simulink library "TM_DynamicModel_Library"  (Simulink 7.8)
settings: Solver=ode45  StartTime=0.0  StopTime=10.0  RelTol=1e-3
undefined symbols (not defined in the file or in its folder): DiscIntNeverNeededParam
libraries: simulink x43, TM_DynamicModel_Library x7
(part 2 of 2)

== system TM_DynamicModel_Library/DM_Eprec_FlgPreCdngAcvMod ==
  Constant : Constant  Value=0
  Eprec_FlgPreCdngAcvMod : Outport
  wires:
  Constant/1 -> Eprec_FlgPreCdngAcvMod/1

== system TM_DynamicModel_Library/DM_Err_ECT_low ==
  Constant : Constant  Value=0
  Err_ECT_low : Outport
  wires:
  Constant/1 -> Err_ECT_low/1

== system TM_DynamicModel_Library/DM_Esig_BmsTpMax ==
  Bms48_Tp : Inport
  Constant : Constant
  Sum : Sum  Inputs=|++
  Esig_BmsTpMax : Outport
  wires:
  Bms48_Tp/1 -> Sum/1
  Sum/1 -> Esig_BmsTpMax/1
  Constant/1 -> Sum/2

== system TM_DynamicModel_Library/DM_Esig_BmsTpMin ==
  Bms48_Tp : Inport
  Constant : Constant
  Sum1 : Sum  Inputs=|-+
  Esig_BmsTpMin : Outport
  wires:
  Bms48_Tp/1 -> Sum1/2
  Constant/1 -> Sum1/1
  Sum1/1 -> Esig_BmsTpMin/1

== system TM_DynamicModel_Library/DM_Esig_BmsTpTar ==
  Constant : Constant  Value=28
  Esig_BmsTpTar : Outport
  wires:
  Constant/1 -> Esig_BmsTpTar/1

== system TM_DynamicModel_Library/DM_FRT_Sens ==
  Constant : Constant  Value=25
  FRT_Sens : Outport
  wires:
  Constant/1 -> FRT_Sens/1

== system TM_DynamicModel_Library/DM_FirstStrt_Mode ==
  Constant : Constant  Value=0
  FirstStrt_Mode : Outport
  wires:
  Constant/1 -> FirstStrt_Mode/1

== system TM_DynamicModel_Library/DM_FirstStrt_Mode_EE ==
  Constant : Constant  Value=0
  FirstStrt_Mode_EE : Outport
  wires:
  Constant/1 -> FirstStrt_Mode_EE/1

== system TM_DynamicModel_Library/DM_Fuel_Temp ==
  Constant : Constant  Value=25
  Fuel_Temp : Outport
  wires:
  Constant/1 -> Fuel_Temp/1

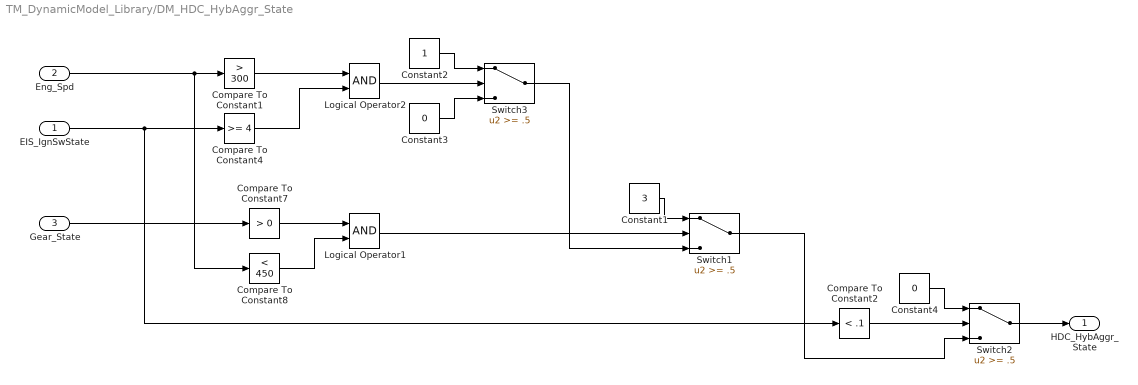
== system TM_DynamicModel_Library/DM_HDC_HybAggr_State ==
  EIS_IgnSwState : Inport
  Eng_Spd : Inport  Port=2
  Gear_State : Inport  Port=3
  Compare To Constant1 : simulink/Logic and Bit Operations/Compare To Constant  relop=>  const=300  OutDataTypeStr=uint8
  Compare To Constant2 : simulink/Logic and Bit Operations/Compare To Constant  relop=<  const=.1  OutDataTypeStr=uint8
  Compare To Constant4 : simulink/Logic and Bit Operations/Compare To Constant  relop=>=  const=4  OutDataTypeStr=uint8
  Compare To Constant7 : simulink/Logic and Bit Operations/Compare To Constant  relop=>  const=0  OutDataTypeStr=uint8
  Compare To Constant8 : simulink/Logic and Bit Operations/Compare To Constant  relop=<  const=450  OutDataTypeStr=uint8
  Constant1 : Constant  Value=3
  Constant2 : Constant
  Constant3 : Constant  Value=0
  Constant4 : Constant  Value=0
  Logical Operator1 : Logic  AllPortsSameDT=off  OutDataTypeStr=boolean
  Logical Operator2 : Logic  AllPortsSameDT=off  OutDataTypeStr=boolean
  Switch1 : Switch  Threshold=.5
  Switch2 : Switch  Threshold=.5
  Switch3 : Switch  Threshold=.5
  HDC_HybAggr_State : Outport
  wires:
  Gear_State/1 -> Compare To Constant7/1
  Eng_Spd/1 -> Compare To Constant8/1, Compare To Constant1/1
  EIS_IgnSwState/1 -> Compare To Constant4/1, Compare To Constant2/1
  Compare To Constant1/1 -> Logical Operator2/1
  Compare To Constant4/1 -> Logical Operator2/2
  Constant2/1 -> Switch3/1
  Constant3/1 -> Switch3/3
  Logical Operator2/1 -> Switch3/2
  Compare To Constant7/1 -> Logical Operator1/1
  Compare To Constant8/1 -> Logical Operator1/2
  Logical Operator1/1 -> Switch1/2
  Constant1/1 -> Switch1/1
  Switch3/1 -> Switch1/3
  Compare To Constant2/1 -> Switch2/2
  Switch1/1 -> Switch2/3
  Switch2/1 -> HDC_HybAggr_State/1
  Constant4/1 -> Switch2/1

== system TM_DynamicModel_Library/DM_HDC_HybSync_State ==
  Eng_Spd : Inport
  Eng_Trq : Inport  Port=2
  Add : Sum
  Add1 : Sum  Inputs=+-
  Add2 : Sum  Inputs=+-
  Constant : Constant  Value=13
  Constant1 : Constant  Value=31
  Constant2 : Constant  Value=0
  Constant3 : Constant  Value=0
  DM_AGC_ASSStop_Mode : TM_DynamicModel_Library/DM_AGC_ASSStop_Mode
  Switch : Switch  Threshold=1
  Switch1 : Switch  Threshold=1
  Unit Delay : UnitDelay  SampleTime=-1
  Unit Delay1 : UnitDelay  SampleTime=-1
  HDC_HybSync_State : Outport
  wires:
  Constant1/1 -> Switch1/1
  Constant2/1 -> Switch1/3
  Switch/1 -> Add/1
  Switch1/1 -> Add/2
  Add/1 -> HDC_HybSync_State/1
  Unit Delay/1 -> Add1/2
  Constant/1 -> Switch/1
  Constant3/1 -> Switch/3
  Add1/1 -> Switch/2
  Unit Delay1/1 -> Add2/1
  Add2/1 -> Switch1/2
  DM_AGC_ASSStop_Mode/1 -> Unit Delay/1, Add1/1, Unit Delay1/1, Add2/2
  Eng_Spd/1 -> DM_AGC_ASSStop_Mode/1
  Eng_Trq/1 -> DM_AGC_ASSStop_Mode/2

== system TM_DynamicModel_Library/DM_HDC_PTReady_Mode ==
  Eng_Spd : Inport
  EIS_IgnSwState : Inport  Port=2
  Compare To Constant : simulink/Logic and Bit Operations/Compare To Constant  relop=<  const=100  OutDataTypeStr=uint8
  Compare To Constant1 : simulink/Logic and Bit Operations/Compare To Constant  relop=>  const=3  OutDataTypeStr=uint8
  Constant : Constant  Value=0
  Constant1 : Constant
  DM_Ign_Mode : Subsystem
  Logical Operator1 : Logic  Operator=OR  Inputs=3  AllPortsSameDT=off  OutDataTypeStr=boolean
  Logical Operator2 : Logic  Operator=NOT  AllPortsSameDT=off  OutDataTypeStr=boolean
  Logical Operator3 : Logic  Operator=NOT  AllPortsSameDT=off  OutDataTypeStr=boolean
  Switch : Switch  Criteria=u2 > Threshold
  HDC_PTReady_Mode : Outport
  wires:
  Eng_Spd/1 -> Compare To Constant/1  "Eng_Spd"
  EIS_IgnSwState/1 -> Compare To Constant1/1, DM_Ign_Mode/1(EIS_IgnSwState)  "EIS_IgnSwState"
  Logical Operator2/1 -> Logical Operator1/2
  Compare To Constant1/1 -> Logical Operator3/1  "IgnSwCAN_Mode"
  Logical Operator3/1 -> Logical Operator1/3
  Switch/1 -> HDC_PTReady_Mode/1
  Logical Operator1/1 -> Switch/2
  Constant1/1 -> Switch/3
  Constant/1 -> Switch/1
  Compare To Constant/1 -> Logical Operator1/1
  DM_Ign_Mode/1(Ign_Mode) -> Logical Operator2/1

== system TM_DynamicModel_Library/DM_HVAC_CoolVlv_Rq ==
  Constant : Constant  Value=0
  HVAC_CoolVlv_Rq : Outport
  wires:
  Constant/1 -> HVAC_CoolVlv_Rq/1

== system TM_DynamicModel_Library/DM_Hepm_PwrMax48VEcm ==
  Constant : Constant  Value=7000
  Hepm_PwrMax48VEcm : Outport
  wires:
  Constant/1 -> Hepm_PwrMax48VEcm/1

== system TM_DynamicModel_Library/DM_Hpmc_StPlgnOpmdDispd ==
  Constant : Constant  Value=3
  Hpmc_StPlgnOpmdDispd : Outport
  wires:
  Constant/1 -> Hpmc_StPlgnOpmdDispd/1

== system TM_DynamicModel_Library/DM_HvacChil_ExpVlvPosnReq ==
  Constant : Constant  Value=0
  HvacChil_ExpVlvPosnReq : Outport
  wires:
  Constant/1 -> HvacChil_ExpVlvPosnReq/1

== system TM_DynamicModel_Library/DM_Hvac_StDefrstAcv ==
  Constant : Constant  Value=0
  Hvac_StDefrstAcv : Outport
  wires:
  Constant/1 -> Hvac_StDefrstAcv/1

== system TM_DynamicModel_Library/DM_IC_Knk_Red_Avg ==
  Constant : Constant  Value=0
  IC_Knk_Red_Avg : Outport
  wires:
  Constant/1 -> IC_Knk_Red_Avg/1

== system TM_DynamicModel_Library/DM_IC_Knk_Red_Avg_Actv ==
  Constant : Constant  Value=0
  IC_Knk_Red_Avg_Actv : Outport
  wires:
  Constant/1 -> IC_Knk_Red_Avg_Actv/1

== system TM_DynamicModel_Library/DM_Idle_Mode_Req ==
  APP : Inport
  Compare To Constant : simulink/Logic and Bit Operations/Compare To Constant  relop=<=  const=3.2  OutDataTypeStr=uint8
  DM_APP_Char_out_ub : Subsystem
  Data Type Conversion : DataTypeConversion
  Idle_Mode_Req : Outport
  wires:
  Data Type Conversion/1 -> Idle_Mode_Req/1
  Compare To Constant/1 -> Data Type Conversion/1
  DM_APP_Char_out_ub/1(APP_Char_out_ub) -> Compare To Constant/1
  APP/1 -> DM_APP_Char_out_ub/1(APP)

== system TM_DynamicModel_Library/DM_IgnSwRun_Mode ==
  EIS_IgnSwState : Inport
  Constant : Constant  Value=4
  Relational Operator : RelationalOperator  Operator===  OutDataTypeStr=boolean
  IgnSwRun_Mode : Outport
  wires:
  Constant/1 -> Relational Operator/2
  EIS_IgnSwState/1 -> Relational Operator/1
  Relational Operator/1 -> IgnSwRun_Mode/1  "IgnSwRun_Mode"

== system TM_DynamicModel_Library/DM_IgnSwStrtr_Mode ==
  EIS_IgnSwState : Inport
  Compare To Constant : simulink/Logic and Bit Operations/Compare To Constant  relop=>  const=4  OutDataTypeStr=uint8
  Compare To Constant1 : simulink/Logic and Bit Operations/Compare To Constant  relop=<  const=6  OutDataTypeStr=uint8
  Data Type Conversion : DataTypeConversion
  Logical Operator : Logic  AllPortsSameDT=off  OutDataTypeStr=boolean
  IgnSwStrtr_Mode : Outport
  wires:
  Data Type Conversion/1 -> IgnSwStrtr_Mode/1
  EIS_IgnSwState/1 -> Compare To Constant/1, Compare To Constant1/1
  Compare To Constant1/1 -> Logical Operator/2
  Compare To Constant/1 -> Logical Operator/1
  Logical Operator/1 -> Data Type Conversion/1

== system TM_DynamicModel_Library/DM_Ign_Mode ==
  EIS_IgnSwState : Inport
  Constant : Constant  Value=3
  Data Type Conversion : DataTypeConversion
  Relational Operator : RelationalOperator  OutDataTypeStr=boolean
  Ign_Mode : Outport
  wires:
  Data Type Conversion/1 -> Ign_Mode/1
  Constant/1 -> Relational Operator/2
  EIS_IgnSwState/1 -> Relational Operator/1
  Relational Operator/1 -> Data Type Conversion/1

== system TM_DynamicModel_Library/DM_Injr_Tp ==
  Constant : Constant  Value=25
  Injr_Tp : Outport
  wires:
  Constant/1 -> Injr_Tp/1

== system TM_DynamicModel_Library/DM_K15 ==
  EIS_IgnSwState : Inport
  Constant : Constant  Value=2
  Data Type Conversion : DataTypeConversion
  Data Type Conversion1 : DataTypeConversion  OutDataTypeStr=uint8
  Relational Operator : RelationalOperator  Operator=>  OutDataTypeStr=boolean
  K15 : Outport
  wires:
  Data Type Conversion1/1 -> Relational Operator/1
  Data Type Conversion/1 -> K15/1
  EIS_IgnSwState/1 -> Data Type Conversion1/1
  Constant/1 -> Relational Operator/2
  Relational Operator/1 -> Data Type Conversion/1  "K15"

== system TM_DynamicModel_Library/DM_LIN_BpShttrGrOvrTemp105_Mode ==
  Constant : Constant  Value=0
  LIN_BpShttrGrOvrTemp105_Mode : Outport
  wires:
  Constant/1 -> LIN_BpShttrGrOvrTemp105_Mode/1

== system TM_DynamicModel_Library/DM_LIN_BpShttrGrOvrTemp_Mode ==
  Constant : Constant  Value=0
  LIN_BpShttrGrOvrTemp_Mode : Outport
  wires:
  Constant/1 -> LIN_BpShttrGrOvrTemp_Mode/1

== system TM_DynamicModel_Library/DM_LIN_BpShttrPosAct_Val ==
  LIN_BpShttrPosReq : Inport
  Unit Delay : UnitDelay  SampleTime=-1
  LIN_BpShttrPosAct_Val : Outport
  wires:
  LIN_BpShttrPosReq/1 -> Unit Delay/1
  Unit Delay/1 -> LIN_BpShttrPosAct_Val/1

== system TM_DynamicModel_Library/DM_LIN_CF_SpdAvg ==
  LIN_CF_Spd_Req : Inport
  Unit Delay : UnitDelay  SampleTime=-1
  LIN_CF_SpdAvg : Outport
  wires:
  LIN_CF_Spd_Req/1 -> Unit Delay/1
  Unit Delay/1 -> LIN_CF_SpdAvg/1

== system TM_DynamicModel_Library/DM_LIN_CP_CAC2TransActlSpd ==
  Tm_BmsClpmpNReq : Inport
  Unit Delay : UnitDelay  SampleTime=-1
  LIN_CP_CAC2TransActlSpd : Outport
  wires:
  Tm_BmsClpmpNReq/1 -> Unit Delay/1
  Unit Delay/1 -> LIN_CP_CAC2TransActlSpd/1

== system TM_DynamicModel_Library/DM_LIN_CP_CAC2TransTp ==
  note: Based on measurements in UDDS and DGR cycles
  Constant : Constant  Value=204
  LIN_CP_CAC2TransTp : Outport
  wires:
  Constant/1 -> LIN_CP_CAC2TransTp/1

== system TM_DynamicModel_Library/DM_LIN_CP_CACTransActlSpd ==
  LIN_CP_CACTransSpd_Req : Inport
  Unit Delay : UnitDelay  SampleTime=-1
  LIN_CP_CACTransActlSpd : Outport
  wires:
  LIN_CP_CACTransSpd_Req/1 -> Unit Delay/1
  Unit Delay/1 -> LIN_CP_CACTransActlSpd/1

== system TM_DynamicModel_Library/DM_LIN_CP_CACTransTgtSpd ==
  LIN_CP_CACTransSpd_Req : Inport
  Delay : Delay  DelayLength=6
  LIN_CP_CACTransTgtSpd : Outport
  wires:
  LIN_CP_CACTransSpd_Req/1 -> Delay/1
  Delay/1 -> LIN_CP_CACTransTgtSpd/1

== system TM_DynamicModel_Library/DM_LIN_CP_CACTransTp ==
  Constant : Constant  Value=45
  LIN_CP_CACTransTp : Outport
  wires:
  Constant/1 -> LIN_CP_CACTransTp/1

== system TM_DynamicModel_Library/DM_LIN_CP_ECP4TransActlSpd ==
  TmPmp_EngClpmpLinReqPwm : Inport
  Unit Delay : UnitDelay  SampleTime=-1
  LIN_CP_ECP4TransActlSpd : Outport
  wires:
  TmPmp_EngClpmpLinReqPwm/1 -> Unit Delay/1
  Unit Delay/1 -> LIN_CP_ECP4TransActlSpd/1

== system TM_DynamicModel_Library/DM_LIN_CP_ECP4TransTp ==
  note: Based on measurements in UDDS and DGR cycles
  Constant : Constant  Value=204
  LIN_CP_ECP4TransTp : Outport
  wires:
  Constant/1 -> LIN_CP_ECP4TransTp/1

== system TM_DynamicModel_Library/DM_LIN_CP_ECP4TransVoltClass ==
  Constant : Constant
  LIN_CP_ECP4TransVoltClass : Outport
  wires:
  Constant/1 -> LIN_CP_ECP4TransVoltClass/1

== system TM_DynamicModel_Library/DM_LIN_CP_ECP4TransVoltStat ==
  Constant : Constant  Value=0
  LIN_CP_ECP4TransVoltStat : Outport
  wires:
  Constant/1 -> LIN_CP_ECP4TransVoltStat/1

== system TM_DynamicModel_Library/DM_LIN_RSV1_CACTransPos_State ==
  LIN_RSV_CACTransPos_State : Inport
  1-D Lookup Table : Lookup_n-D  NumberOfTableDimensions=1  BreakpointsForDimension1=[3,4,5,6,7,8]  Table=[1308,1496,1688,1876,1972,2068]  RndMeth=Simplest  InputSameDT=on
  LIN_RSV1_CACTransPos_State : Outport
  wires:
  LIN_RSV_CACTransPos_State/1 -> 1-D Lookup Table/1
  1-D Lookup Table/1 -> LIN_RSV1_CACTransPos_State/1

== system TM_DynamicModel_Library/DM_LIN_RSV_CACTransMove_State ==
  Constant : Constant  Value=0
  LIN_RSV_CACTransMove_State : Outport
  wires:
  Constant/1 -> LIN_RSV_CACTransMove_State/1

== system TM_DynamicModel_Library/DM_LIN_ShttrPosAct_Val ==
  LIN_ShttrPosReq : Inport
  Unit Delay : UnitDelay  SampleTime=-1
  LIN_ShttrPosAct_Val : Outport
  wires:
  LIN_ShttrPosReq/1 -> Unit Delay/1
  Unit Delay/1 -> LIN_ShttrPosAct_Val/1

== system TM_DynamicModel_Library/DM_LIN_ShttrPosMove_State ==
  Constant : Constant  Value=0
  LIN_ShttrPosMove_State : Outport
  wires:
  Constant/1 -> LIN_ShttrPosMove_State/1

== system TM_DynamicModel_Library/DM_MTX_Mode ==
  Constant : Constant  Value=0
  MTX_Mode : Outport
  wires:
  Constant/1 -> MTX_Mode/1

== system TM_DynamicModel_Library/DM_Net_EBoost_CurrCons ==
  Constant : Constant  Value=0
  Net_EBoost_CurrCons : Outport
  wires:
  Constant/1 -> Net_EBoost_CurrCons/1

== system TM_DynamicModel_Library/DM_Net_Eboost_PCB_Temp ==
  note: 25-04-2017
      | Eboost PCB temp is assumed to be higher than the inlet coolant temperature by 5 degC
  CacInTp_Tp : Inport
  Constant : Constant  Value=5
  Sum : Sum  Inputs=|++
  Net_Eboost_PCB_Temp : Outport
  wires:
  Constant/1 -> Sum/2
  Sum/1 -> Net_Eboost_PCB_Temp/1
  CacInTp_Tp/1 -> Sum/1

== system TM_DynamicModel_Library/DM_Odo_Abs_HighRes ==
  note: Sample Time = 0.1s
  Veh_Spd : Inport
  Gain : Gain  Gain=1/3600
  Initial Odo value : Constant  Value=0
  Integrator : Integrator  InitialConditionSource=external
  Odo_Abs_HighRes : Outport
  wires:
  Veh_Spd/1 -> Gain/1
  Initial Odo value/1 -> Integrator/2
  Integrator/1 -> Odo_Abs_HighRes/1
  Gain/1 -> Integrator/1

== system TM_DynamicModel_Library/DM_Odo_Abs_Long ==
  note: Sample Time = 0.1s
  Veh_Spd : Inport
  Gain : Gain  Gain=1/3600
  Initial Odo value : Constant  Value=0
  Integrator : Integrator  InitialConditionSource=external
  Odo_Abs_Long : Outport
  wires:
  Gain/1 -> Integrator/1
  Integrator/1 -> Odo_Abs_Long/1
  Initial Odo value/1 -> Integrator/2
  Veh_Spd/1 -> Gain/1

== system TM_DynamicModel_Library/DM_Pnct48V_VoltMinThdShutDwnEcm ==
  Constant : Constant  Value=37
  Pnct48V_VoltMinThdShutDwnEcm : Outport
  wires:
  Constant/1 -> Pnct48V_VoltMinThdShutDwnEcm/1

== system TM_DynamicModel_Library/DM_Pnct48_HtCoolPwrRq ==
  Constant : Constant  Value=0
  Pnct48_HtCoolPwrRq : Outport
  wires:
  Constant/1 -> Pnct48_HtCoolPwrRq/1

== system TM_DynamicModel_Library/DM_Pnct48_PwrPackBatTempMax ==
  Bms48_Tp : Inport
  Constant : Constant
  Sum : Sum  Inputs=|++
  Pnct48_PwrPackBatTempMax : Outport
  wires:
  Bms48_Tp/1 -> Sum/1
  Sum/1 -> Pnct48_PwrPackBatTempMax/1
  Constant/1 -> Sum/2

== system TM_DynamicModel_Library/DM_Pnct48_PwrPackBatTempMin ==
  Bms48_Tp : Inport
  Constant : Constant
  Sum1 : Sum  Inputs=|-+
  Pnct48_PwrPackBatTempMin : Outport
  wires:
  Bms48_Tp/1 -> Sum1/2
  Constant/1 -> Sum1/1
  Sum1/1 -> Pnct48_PwrPackBatTempMin/1

== system TM_DynamicModel_Library/DM_RsvBms_PosnAct ==
  Constant : Constant  Value=0
  RsvBms_PosnAct : Outport
  wires:
  Constant/1 -> RsvBms_PosnAct/1

== system TM_DynamicModel_Library/DM_RsvLoTpCcr_PosnAvlFlg ==
  LIN_RSV_CACTransPos_State : Inport
  Add : Sum
  Constant : Constant
  Constant1 : Constant  Value=5
  Constant2 : Constant
  Constant3 : Constant  Value=5
  Data Type Conversion : DataTypeConversion  OutDataTypeStr=int8
  Data Type Conversion1 : DataTypeConversion
  Logical Operator : Logic  Operator=NOT  AllPortsSameDT=off  OutDataTypeStr=boolean
  Memory : Memory  X0=1  InheritSampleTime=on
  Relational Operator : RelationalOperator  Operator=~=  OutDataTypeStr=boolean
  Relational Operator1 : RelationalOperator  Operator=<=  OutDataTypeStr=boolean
  Switch : Switch  Criteria=u2 > Threshold
  Switch1 : Switch  Criteria=u2 > Threshold
  Unit Delay : UnitDelay  SampleTime=-1
  RsvLoTpCcr_PosnAvlFlg : Outport
  wires:
  Data Type Conversion1/1 -> RsvLoTpCcr_PosnAvlFlg/1
  LIN_RSV_CACTransPos_State/1 -> Data Type Conversion/1
  Unit Delay/1 -> Relational Operator/2
  Relational Operator/1 -> Switch1/2
  Data Type Conversion/1 -> Relational Operator/1, Unit Delay/1
  Constant3/1 -> Switch1/3
  Switch1/1 -> Add/1
  Switch/1 -> Memory/1
  Constant2/1 -> Switch/3
  Relational Operator1/1 -> Switch/2, Logical Operator/1
  Constant1/1 -> Relational Operator1/2
  Add/1 -> Switch/1, Relational Operator1/1
  Constant/1 -> Add/2
  Memory/1 -> Switch1/1
  Logical Operator/1 -> Data Type Conversion1/1

== system TM_DynamicModel_Library/DM_ScrcmDos_THeatrPmpAftRunReq ==
  Constant : Constant  Value=0
  ScrcmDos_THeatrPmpAftRunReq : Outport
  wires:
  Constant/1 -> ScrcmDos_THeatrPmpAftRunReq/1

== system TM_DynamicModel_Library/DM_TCC_Spd ==
  Eng_Spd : Inport
  Compare To Constant : simulink/Logic and Bit Operations/Compare To Constant  relop=>=  const=550  OutDataTypeStr=uint8
  Constant : Constant  Value=0
  Switch : Switch  Criteria=u2 > Threshold
  TCC_Spd : Outport
  wires:
  Switch/1 -> TCC_Spd/1
  Eng_Spd/1 -> Compare To Constant/1, Switch/1
  Compare To Constant/1 -> Switch/2
  Constant/1 -> Switch/3

== system TM_DynamicModel_Library/DM_Tc_FlgTpCrit ==
  note: 25-04-2017: Setting this a zero
  Constant : Constant  Value=0
  Tc_FlgTpCrit : Outport
  wires:
  Constant/1 -> Tc_FlgTpCrit/1

== system TM_DynamicModel_Library/DM_ThrOutPSnsr_P ==
  Constant : Constant  Value=0
  ThrOutPSnsr_P : Outport
  wires:
  Constant/1 -> ThrOutPSnsr_P/1

== system TM_DynamicModel_Library/DM_TmBmsCcr_SnsrTpRaw ==
  TmBmsCcr_SnsrTp : Inport
  1-D Lookup Table:  TmBmsCcr_SnsrTpActVal_L : Lookup_n-D  NumberOfTableDimensions=1  BreakpointsForDimension1="[-40.0000  -32.3750  -22.7500  -13.7500   -5.0000    5.3750   16.7500   29.2500   50.7500   65.0000   77.3750   93.5000  109.1250  125.0000  141.6250  150.0000]"  IndexSearchMethod=Linear search  Table="[ 4.9451    4.9109    4.8376    4.7326    4.5702    4.3236    3.9133    3.3785    2.3419    1.7265    1.2845    0.8645    0.5885    0.4054    0.2772    0.2332]"  RndMeth=Simplest  InputSameDT=on
  TmBmsCcr_SnsrTpRaw : Outport
  wires:
  TmBmsCcr_SnsrTp/1 -> 1-D Lookup Table:  TmBmsCcr_SnsrTpActVal_L/1
  1-D Lookup Table:  TmBmsCcr_SnsrTpActVal_L/1 -> TmBmsCcr_SnsrTpRaw/1

== system TM_DynamicModel_Library/DM_TmBmsPSnsrChil_VoltRaw ==
  Constant : Constant  Value=4.5
  TmBmsPSnsrChil_VoltRaw : Outport
  wires:
  Constant/1 -> TmBmsPSnsrChil_VoltRaw/1

== system TM_DynamicModel_Library/DM_TmBmsTpSnsrChil_ActVoltRaw ==
  Constant : Constant  Value=4.5
  TmBmsTpSnsrChil_ActVoltRaw : Outport
  wires:
  Constant/1 -> TmBmsTpSnsrChil_ActVoltRaw/1

== system TM_DynamicModel_Library/DM_TmGbOil_PredCtlAcvnFlg ==
  Constant : Constant  Value=0
  TmGbOil_PredCtlAcvnFlg : Outport
  wires:
  Constant/1 -> TmGbOil_PredCtlAcvnFlg/1

== system TM_DynamicModel_Library/DM_TmLoTpCcr2_FillLvlVoltRaw ==
  note: Sample Time = 0.1s
  AGB_WaterLevel : Inport
  %_to_Volt : Gain  Gain=5/100
  TmLoTpCcr2_FillLvlVoltRaw : Outport
  wires:
  %_to_Volt/1 -> TmLoTpCcr2_FillLvlVoltRaw/1
  AGB_WaterLevel/1 -> %_to_Volt/1

== system TM_DynamicModel_Library/DM_TmLoTpCcr_SnsrTpRaw ==
  TmLtCcr_SnsrTpAct : Inport
  "1-D Lookup Table: TmLtCcr_SnsrTpActVal_L " : Lookup_n-D  NumberOfTableDimensions=1  BreakpointsForDimension1="[-40.0000  -32.3750  -22.7500  -13.7500   -5.0000    5.3750   16.7500   29.2500   50.7500   65.0000   77.3750   93.5000  109.1250  125.0000  141.6250  150.0000]"  IndexSearchMethod=Linear search  Table="[4.9451    4.9109    4.8376    4.7326    4.5702    4.3236    3.9133    3.3785    2.3419    1.7265    1.2845    0.8645    0.5885    0.4054    0.2772    0.2332]"  RndMeth=Simplest  InputSameDT=on
  TmLoTpCcr_SnsrTpRaw : Outport
  wires:
  TmLtCcr_SnsrTpAct/1 -> "1-D Lookup Table: TmLtCcr_SnsrTpActVal_L "/1
  "1-D Lookup Table: TmLtCcr_SnsrTpActVal_L "/1 -> TmLoTpCcr_SnsrTpRaw/1

== system TM_DynamicModel_Library/DM_TmLt2Chil_HeatTrfAdpnEnaFlgDly ==
  Constant : Constant
  TmLt2Chil_HeatTrfAdpnEnaFlgDly : Outport
  wires:
  Constant/1 -> TmLt2Chil_HeatTrfAdpnEnaFlgDly/1

== system TM_DynamicModel_Library/DM_TmLt2CoolRedn_HeatTrfAdpnEnaFlgDly ==
  Constant : Constant  Value=0
  TmLt2CoolRedn_HeatTrfAdpnEnaFlgDly : Outport
  wires:
  Constant/1 -> TmLt2CoolRedn_HeatTrfAdpnEnaFlgDly/1

== system TM_DynamicModel_Library/DM_TmPredHvBatCoolg_TpSpAcvFlg ==
  Constant : Constant  Value=0
  TmPredHvBatCoolg_TpSpAcvFlg : Outport
  wires:
  Constant/1 -> TmPredHvBatCoolg_TpSpAcvFlg/1

== system TM_DynamicModel_Library/DM_TmPredQckwnsBatCoolt_BatTpSp ==
  Constant : Constant  Value=0
  TmPredQckwnsBatCoolt_BatTpSp : Outport
  wires:
  Constant/1 -> TmPredQckwnsBatCoolt_BatTpSp/1

== system TM_DynamicModel_Library/DM_Trans_OilTempHigh_Mode ==
  Constant : Constant  Value=0
  Trans_OilTempHigh_Mode : Outport
  wires:
  Constant/1 -> Trans_OilTempHigh_Mode/1

== system TM_DynamicModel_Library/DM_TrqSetIgn_Mode_Req ==
  Constant : Constant  Value=0
  TrqSetIgn_Mode_Req : Outport
  wires:
  Constant/1 -> TrqSetIgn_Mode_Req/1

== system TM_DynamicModel_Library/DM_TrqSetRes_Mode_Req ==
  Constant : Constant  Value=0
  TrqSetRes_Mode_Req : Outport
  wires:
  Constant/1 -> TrqSetRes_Mode_Req/1

== system TM_DynamicModel_Library/DM_VehMass_Wght_Pred ==
  Constant : Constant  Value=1974
  VehMass_Wght_Pred : Outport
  wires:
  Constant/1 -> VehMass_Wght_Pred/1

== system TM_DynamicModel_Library/DM_ag_CamsftExhSp ==
  Constant : Constant  Value=0
  ag_CamsftExhSp : Outport
  wires:
  Constant/1 -> ag_CamsftExhSp/1

== system TM_DynamicModel_Library/DM_ag_CamsftIntkSp ==
  Constant : Constant  Value=0
  ag_CamsftIntkSp : Outport
  wires:
  Constant/1 -> ag_CamsftIntkSp/1

== system TM_DynamicModel_Library/DM_nst08 ==
  Eng_Spd : Inport
  Data Type Conversion : DataTypeConversion
  NISTV08 : PreLookup  BreakpointsData="[500.0000000000000000   1000.0000000000000000   1500.0000000000000000   2000.0000000000000000   3000.0000000000000000   4000.0000000000000000  4800.0000000000000000   6000.0000000000000000]"  OutputOnlyTheIndex=on
  nst08 : Outport
  wires:
  Eng_Spd/1 -> NISTV08/1
  NISTV08/1 -> Data Type Conversion/1
  Data Type Conversion/1 -> nst08/1

== system TM_DynamicModel_Library/DM_AGC_DTREngCutOff_Mode/DM_Ign_Mode ==
  EIS_IgnSwState : Inport
  Constant : Constant  Value=3
  Relational Operator : RelationalOperator  OutDataTypeStr=boolean
  Ign_Mode : Outport
  wires:
  Constant/1 -> Relational Operator/2
  EIS_IgnSwState/1 -> Relational Operator/1
  Relational Operator/1 -> Ign_Mode/1

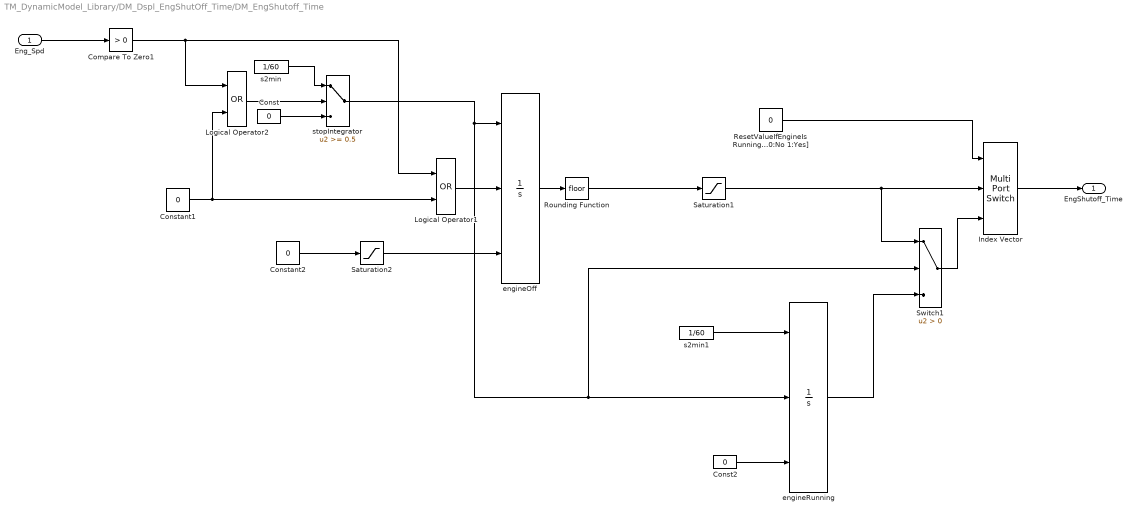
== system TM_DynamicModel_Library/DM_Dspl_EngShutOff_Time/DM_EngShutoff_Time ==
  Eng_Spd : Inport
  Compare To Zero1 : simulink/Logic and Bit Operations/Compare To Zero  relop=>  OutDataTypeStr=uint8
  Const : Constant  Value=0
  Const2 : Constant  Value=0
  Constant1 : Constant  Value=0
  Constant2 : Constant  Value=0
  Index Vector : MultiPortSwitch  DataPortOrder=Zero-based contiguous  Inputs=2  zeroidx=on
  Logical Operator1 : Logic  Operator=OR  AllPortsSameDT=off
  Logical Operator2 : Logic  Operator=OR  AllPortsSameDT=off
  ResetValueIfEngineIsRunning [0:No 1:Yes] : Constant  Value=0
  Rounding Function : Rounding
  Saturation1 : Saturate  UpperLimit=4095  LowerLimit=0
  Saturation2 : Saturate  UpperLimit=4095  LowerLimit=0  OutDataTypeStr=double
  Switch1 : Switch  Criteria=u2 > Threshold  SaturateOnIntegerOverflow=on
  engineOff : Integrator  ExternalReset=falling  InitialConditionSource=external
  engineRunning : Integrator  ExternalReset=falling  InitialConditionSource=external
  s2min : Constant  Value=1/60
  s2min1 : Constant  Value=1/60
  stopIntegrator : Switch  Threshold=0.5  SaturateOnIntegerOverflow=on
  EngShutoff_Time : Outport
  wires:
  Compare To Zero1/1 -> Logical Operator2/1, Logical Operator1/1
  Eng_Spd/1 -> Compare To Zero1/1
  s2min1/1 -> engineRunning/1
  Const2/1 -> engineRunning/3
  engineRunning/1 -> Switch1/3
  Switch1/1 -> Index Vector/3
  ResetValueIfEngineIsRunning [0:No 1:Yes]/1 -> Index Vector/1
  Index Vector/1 -> EngShutoff_Time/1
  Const/1 -> stopIntegrator/3
  s2min/1 -> stopIntegrator/1
  stopIntegrator/1 -> engineRunning/2, Switch1/2, engineOff/1
  Constant1/1 -> Logical Operator1/2, Logical Operator2/2
  Logical Operator1/1 -> engineOff/2
  Saturation1/1 -> Switch1/1, Index Vector/2
  engineOff/1 -> Rounding Function/1
  Rounding Function/1 -> Saturation1/1
  Logical Operator2/1 -> stopIntegrator/2
  Saturation2/1 -> engineOff/3
  Constant2/1 -> Saturation2/1

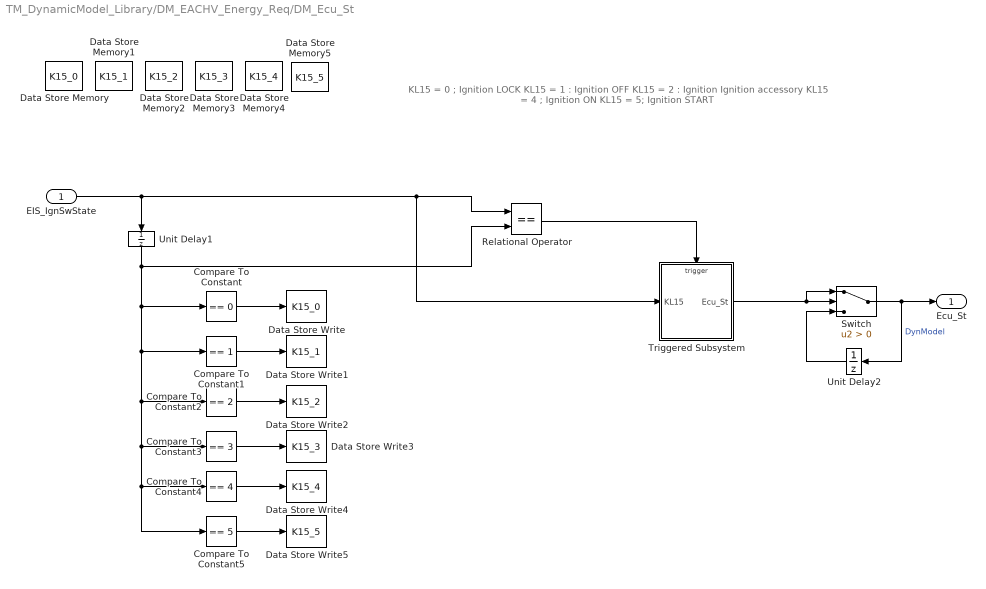
== system TM_DynamicModel_Library/DM_EACHV_Energy_Req/DM_Ecu_St ==
  note: KL15 = 0 ; Ignition LOCK
      | KL15 = 1 : Ignition OFF
      | KL15 = 2 : Ignition Ignition accessory
      | KL15 = 4 ; Ignition ON
      | KL15 = 5; Ignition START
  EIS_IgnSwState : Inport  SampleTime=0.1
  Compare To Constant : simulink/Logic and Bit Operations/Compare To Constant  relop===  const=0  OutDataTypeStr=uint8
  Compare To Constant1 : simulink/Logic and Bit Operations/Compare To Constant  relop===  const=1  OutDataTypeStr=uint8
  Compare To Constant2 : simulink/Logic and Bit Operations/Compare To Constant  relop===  const=2  OutDataTypeStr=uint8
  Compare To Constant3 : simulink/Logic and Bit Operations/Compare To Constant  relop===  const=3  OutDataTypeStr=uint8
  Compare To Constant4 : simulink/Logic and Bit Operations/Compare To Constant  relop===  const=4  OutDataTypeStr=uint8
  Compare To Constant5 : simulink/Logic and Bit Operations/Compare To Constant  relop===  const=5  OutDataTypeStr=uint8
  Data Store Memory : DataStoreMemory  DataStoreName=K15_0  ReadBeforeWriteMsg=warning  WriteAfterWriteMsg=warning  WriteAfterReadMsg=warning
  Data Store Memory1 : DataStoreMemory  DataStoreName=K15_1  ReadBeforeWriteMsg=warning  WriteAfterWriteMsg=warning  WriteAfterReadMsg=warning
  Data Store Memory2 : DataStoreMemory  DataStoreName=K15_2  ReadBeforeWriteMsg=warning  WriteAfterWriteMsg=warning  WriteAfterReadMsg=warning
  Data Store Memory3 : DataStoreMemory  DataStoreName=K15_3  ReadBeforeWriteMsg=warning  WriteAfterWriteMsg=warning  WriteAfterReadMsg=warning
  Data Store Memory4 : DataStoreMemory  DataStoreName=K15_4  ReadBeforeWriteMsg=warning  WriteAfterWriteMsg=warning  WriteAfterReadMsg=warning
  Data Store Memory5 : DataStoreMemory  DataStoreName=K15_5  ReadBeforeWriteMsg=warning  WriteAfterWriteMsg=warning  WriteAfterReadMsg=warning
  Data Store Write : DataStoreWrite  DataStoreName=K15_0
  Data Store Write1 : DataStoreWrite  DataStoreName=K15_1
  Data Store Write2 : DataStoreWrite  DataStoreName=K15_2
  Data Store Write3 : DataStoreWrite  DataStoreName=K15_3
  Data Store Write4 : DataStoreWrite  DataStoreName=K15_4
  Data Store Write5 : DataStoreWrite  DataStoreName=K15_5
  Relational Operator : RelationalOperator  Operator===  OutDataTypeStr=boolean
  Switch : Switch  Criteria=u2 > Threshold
  Triggered Subsystem : Subsystem  TreatAsAtomicUnit=on
  Unit Delay1 : UnitDelay  SampleTime=-1
  Unit Delay2 : UnitDelay  SampleTime=-1
  Ecu_St : Outport  SampleTime=0.1
  wires:
  Unit Delay2/1 -> Switch/3
  Switch/1 -> Ecu_St/1, Unit Delay2/1  "DynModel"
  Unit Delay1/1 -> Relational Operator/2, Compare To Constant/1, Compare To Constant1/1, Compare To Constant2/1, Compare To Constant3/1, Compare To Constant5/1, Compare To Constant4/1
  Triggered Subsystem/1(Ecu_St) -> Switch/1, Switch/2
  Relational Operator/1 -> Triggered Subsystem/Trigger
  Compare To Constant5/1 -> Data Store Write5/1
  Compare To Constant4/1 -> Data Store Write4/1
  Compare To Constant3/1 -> Data Store Write3/1
  Compare To Constant2/1 -> Data Store Write2/1
  EIS_IgnSwState/1 -> Unit Delay1/1, Triggered Subsystem/1(KL15), Relational Operator/1
  Compare To Constant1/1 -> Data Store Write1/1
  Compare To Constant/1 -> Data Store Write/1

== system TM_DynamicModel_Library/DM_EACHV_SwClosed/DM_ESIG_BMS_Switch_State ==
  EIS_IgnSwState : Inport
  Compare To Constant : simulink/Logic and Bit Operations/Compare To Constant  relop=<  const=1.0  OutDataTypeStr=uint8
  Data Type Conversion : DataTypeConversion
  Delay : Delay  DelayLength=15000  InitialCondition=2  SampleTime=0.1
  Gain : Gain  Gain=2
  Logical Operator : Logic  Operator=NOT  AllPortsSameDT=off  OutDataTypeStr=boolean
  ESIG_BMS_Switch_State : Outport
  wires:
  Data Type Conversion/1 -> ESIG_BMS_Switch_State/1
  EIS_IgnSwState/1 -> Compare To Constant/1
  Delay/1 -> Data Type Conversion/1
  Compare To Constant/1 -> Logical Operator/1
  Logical Operator/1 -> Gain/1
  Gain/1 -> Delay/1

== system TM_DynamicModel_Library/DM_EACHV_SwOpen/DM_ESIG_BMS_Switch_State ==
  EIS_IgnSwState : Inport
  Compare To Constant : simulink/Logic and Bit Operations/Compare To Constant  relop=<  const=1.0  OutDataTypeStr=uint8
  Delay : Delay  DelayLength=15000  InitialCondition=2  SampleTime=0.1
  Gain : Gain  Gain=2
  Logical Operator : Logic  Operator=NOT  AllPortsSameDT=off  OutDataTypeStr=boolean
  ESIG_BMS_Switch_State : Outport
  wires:
  EIS_IgnSwState/1 -> Compare To Constant/1
  Delay/1 -> ESIG_BMS_Switch_State/1
  Compare To Constant/1 -> Logical Operator/1
  Logical Operator/1 -> Gain/1
  Gain/1 -> Delay/1

== system TM_DynamicModel_Library/DM_ECU_Ign_Time/Counter_RE ==
  Enable : Inport
  Reset : Inport  Port=2
  InitVal : Inport  Port=3
  Add1 : Sum
  Constant1 : Constant
  Switch2 : Switch  Threshold=1
  Switch3 : Switch  Threshold=1
  Unit Delay3 : UnitDelay  SampleTime=-1
  y : Outport  InitialOutput=0
  wires:
  Switch3/1 -> y/1, Unit Delay3/1  "c_k"
  Unit Delay3/1 -> Switch2/3, Add1/1  "c_km1"
  Constant1/1 -> Add1/2
  Add1/1 -> Switch2/1
  Enable/1 -> Switch2/2
  InitVal/1 -> Switch3/1
  Switch2/1 -> Switch3/3
  Reset/1 -> Switch3/2

== system TM_DynamicModel_Library/DM_ECU_Ign_Time/EdgeBi ==
  u : Inport
  R : Inport  Port=2
  IV : Inport  Port=3
  Relational Operator : RelationalOperator  Operator=~=  OutDataTypeStr=boolean
  Switch2 : Switch  Threshold=1
  Unit Delay3 : UnitDelay  SampleTime=-1
  y : Outport  InitialOutput=0
  wires:
  Switch2/1 -> Relational Operator/2
  Relational Operator/1 -> y/1  "y_k"
  u/1 -> Unit Delay3/1, Relational Operator/1
  R/1 -> Switch2/2
  Unit Delay3/1 -> Switch2/3  "u_km1"
  IV/1 -> Switch2/1

== system TM_DynamicModel_Library/DM_ECU_Ign_Time/IgnSwRun_Mode ==
  IgnKeyPosition : Inport
  Constant : Constant  Value=4
  Relational Operator : RelationalOperator  Operator===  OutDataTypeStr=boolean
  IgnSwRun_Mode : Outport
  wires:
  Constant/1 -> Relational Operator/2
  IgnKeyPosition/1 -> Relational Operator/1
  Relational Operator/1 -> IgnSwRun_Mode/1  "IgnSwRun_Mode"

== system TM_DynamicModel_Library/DM_EM2_StMachn_State/Subsystem2 ==
  In1 : Inport
  Enable : EnablePort
  Out1 : Outport
  wires:
  In1/1 -> Out1/1

== system TM_DynamicModel_Library/DM_EM2_Temp/Subsystem ==
  V : Inport
  I : Inport  Port=2
  Trq : Inport  Port=3
  Spd : Inport  Port=4
  Abs1 : Abs
  Abs2 : Abs
  Add : Sum  Inputs=+-
  Product : Product  RndMeth=Zero
  Product1 : Product  RndMeth=Zero
  dQ : Outport
  wires:
  Product/1 -> Abs1/1
  Product1/1 -> Add/2
  Add/1 -> Abs2/1
  V/1 -> Product/1
  I/1 -> Product/2
  Trq/1 -> Product1/1
  Spd/1 -> Product1/2
  Abs2/1 -> dQ/1
  Abs1/1 -> Add/1

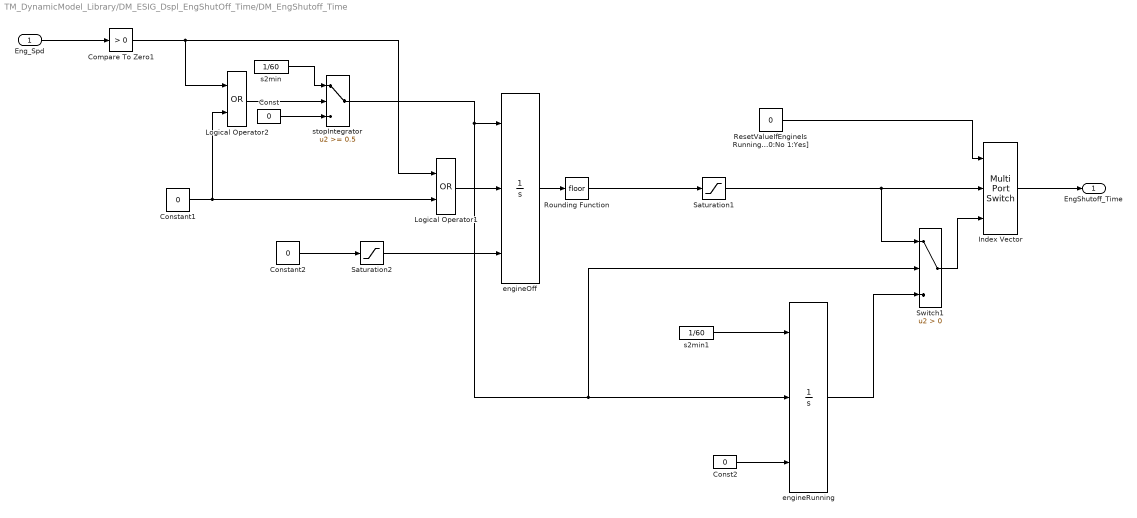
== system TM_DynamicModel_Library/DM_ESIG_Dspl_EngShutOff_Time/DM_EngShutoff_Time ==
  Eng_Spd : Inport
  Compare To Zero1 : simulink/Logic and Bit Operations/Compare To Zero  relop=>  OutDataTypeStr=uint8
  Const : Constant  Value=0
  Const2 : Constant  Value=0
  Constant1 : Constant  Value=0
  Constant2 : Constant  Value=0
  Index Vector : MultiPortSwitch  DataPortOrder=Zero-based contiguous  Inputs=2  zeroidx=on
  Logical Operator1 : Logic  Operator=OR  AllPortsSameDT=off
  Logical Operator2 : Logic  Operator=OR  AllPortsSameDT=off
  ResetValueIfEngineIsRunning [0:No 1:Yes] : Constant  Value=0
  Rounding Function : Rounding
  Saturation1 : Saturate  UpperLimit=4095  LowerLimit=0
  Saturation2 : Saturate  UpperLimit=4095  LowerLimit=0  OutDataTypeStr=double
  Switch1 : Switch  Criteria=u2 > Threshold  SaturateOnIntegerOverflow=on
  engineOff : Integrator  ExternalReset=falling  InitialConditionSource=external
  engineRunning : Integrator  ExternalReset=falling  InitialConditionSource=external
  s2min : Constant  Value=1/60
  s2min1 : Constant  Value=1/60
  stopIntegrator : Switch  Threshold=0.5  SaturateOnIntegerOverflow=on
  EngShutoff_Time : Outport
  wires:
  Compare To Zero1/1 -> Logical Operator2/1, Logical Operator1/1
  Eng_Spd/1 -> Compare To Zero1/1
  s2min1/1 -> engineRunning/1
  Const2/1 -> engineRunning/3
  engineRunning/1 -> Switch1/3
  Switch1/1 -> Index Vector/3
  ResetValueIfEngineIsRunning [0:No 1:Yes]/1 -> Index Vector/1
  Index Vector/1 -> EngShutoff_Time/1
  Const/1 -> stopIntegrator/3
  s2min/1 -> stopIntegrator/1
  stopIntegrator/1 -> engineRunning/2, Switch1/2, engineOff/1
  Constant1/1 -> Logical Operator1/2, Logical Operator2/2
  Logical Operator1/1 -> engineOff/2
  Saturation1/1 -> Switch1/1, Index Vector/2
  engineOff/1 -> Rounding Function/1
  Rounding Function/1 -> Saturation1/1
  Logical Operator2/1 -> stopIntegrator/2
  Saturation2/1 -> engineOff/3
  Constant2/1 -> Saturation2/1

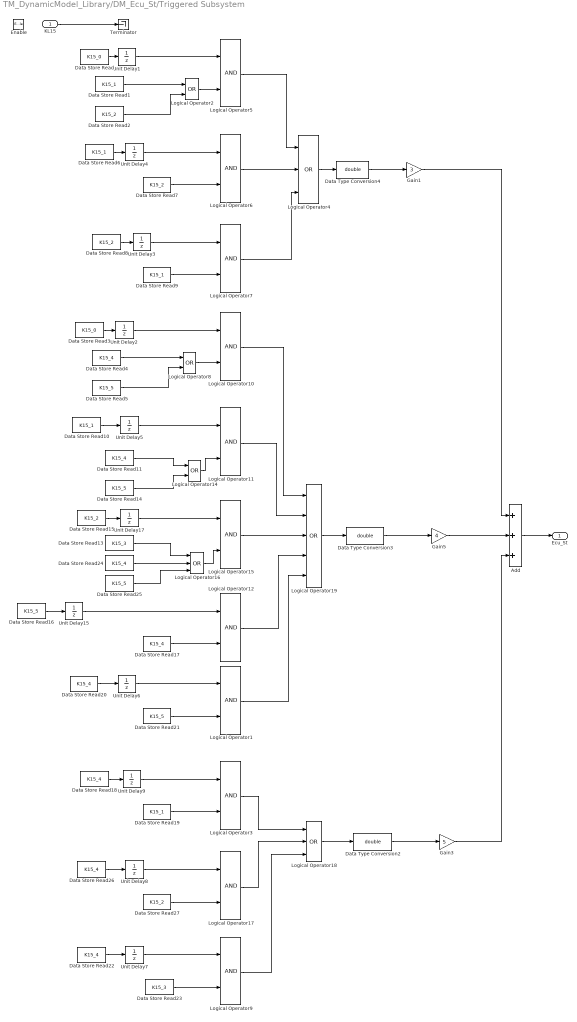
== system TM_DynamicModel_Library/DM_Ecu_St/Triggered Subsystem ==
  KL15 : Inport
  Enable : EnablePort
  Add : Sum  Inputs=+++
  Data Store Read : DataStoreRead  DataStoreName=K15_0
  Data Store Read{1,6,9..10,19} (5 alike) : DataStoreRead  DataStoreName=K15_1
  Data Store Read{4,11,17..18,20,22,24,26} (8 alike) : DataStoreRead  DataStoreName=K15_4
  Data Store Read13 : DataStoreRead  DataStoreName=K15_3
  Data Store Read{5,14,16,21,25} (5 alike) : DataStoreRead  DataStoreName=K15_5
  Data Store Read{2,7..8,15,27} (5 alike) : DataStoreRead  DataStoreName=K15_2
  Data Store Read23 : DataStoreRead  DataStoreName=K15_3
  Data Store Read3 : DataStoreRead  DataStoreName=K15_0
  Data Type Conversion2 : DataTypeConversion  OutDataTypeStr=double
  Data Type Conversion3 : DataTypeConversion  OutDataTypeStr=double
  Data Type Conversion4 : DataTypeConversion  OutDataTypeStr=double
  Gain1 : Gain  Gain=3
  Gain3 : Gain  Gain=5
  Gain5 : Gain  Gain=4
  Logical Operator{1,3,5..7,9..12,15,17} (11 alike) : Logic  AllPortsSameDT=off  OutDataTypeStr=boolean
  Logical Operator14 : Logic  Operator=OR  AllPortsSameDT=off  OutDataTypeStr=boolean
  Logical Operator16 : Logic  Operator=OR  Inputs=3  AllPortsSameDT=off  OutDataTypeStr=boolean
  Logical Operator18 : Logic  Operator=OR  Inputs=3  AllPortsSameDT=off  OutDataTypeStr=boolean
  Logical Operator19 : Logic  Operator=OR  Inputs=5  AllPortsSameDT=off  OutDataTypeStr=boolean
  Logical Operator2 : Logic  Operator=OR  AllPortsSameDT=off  OutDataTypeStr=boolean
  Logical Operator4 : Logic  Operator=OR  Inputs=3  AllPortsSameDT=off  OutDataTypeStr=boolean
  Logical Operator8 : Logic  Operator=OR  AllPortsSameDT=off  OutDataTypeStr=boolean
  Terminator : Terminator
  Unit Delay{1..9,15,17} (11 alike) : UnitDelay  SampleTime=-1
  Ecu_St : Outport
  wires:
  Logical Operator9/1 -> Logical Operator18/3
  Unit Delay7/1 -> Logical Operator9/1
  Data Store Read22/1 -> Unit Delay7/1
  Data Store Read23/1 -> Logical Operator9/2
  Data Store Read25/1 -> Logical Operator16/3
  Data Store Read24/1 -> Logical Operator16/2
  Data Store Read13/1 -> Logical Operator16/1
  Unit Delay8/1 -> Logical Operator17/1
  Unit Delay9/1 -> Logical Operator3/1
  Unit Delay6/1 -> Logical Operator1/1
  Unit Delay15/1 -> Logical Operator12/1
  Unit Delay17/1 -> Logical Operator15/1
  Unit Delay5/1 -> Logical Operator11/1
  Unit Delay2/1 -> Logical Operator10/1
  Unit Delay3/1 -> Logical Operator7/1
  Unit Delay4/1 -> Logical Operator6/1
  Unit Delay1/1 -> Logical Operator5/1
  Logical Operator1/1 -> Logical Operator19/5
  Logical Operator12/1 -> Logical Operator19/4
  Logical Operator15/1 -> Logical Operator19/3
  Logical Operator11/1 -> Logical Operator19/2
  Logical Operator10/1 -> Logical Operator19/1
  Data Store Read18/1 -> Unit Delay9/1
  Data Store Read19/1 -> Logical Operator3/2
  Data Type Conversion2/1 -> Gain3/1
  Data Store Read/1 -> Unit Delay1/1
  Data Store Read6/1 -> Unit Delay4/1
  Data Store Read8/1 -> Unit Delay3/1
  Data Store Read9/1 -> Logical Operator7/2
  Logical Operator5/1 -> Logical Operator4/1
  Logical Operator6/1 -> Logical Operator4/2
  Logical Operator7/1 -> Logical Operator4/3
  Logical Operator4/1 -> Data Type Conversion4/1
  Data Store Read16/1 -> Unit Delay15/1
  Data Store Read17/1 -> Logical Operator12/2
  Data Type Conversion3/1 -> Gain5/1
  Data Type Conversion4/1 -> Gain1/1
  Data Store Read7/1 -> Logical Operator6/2
  Logical Operator2/1 -> Logical Operator5/2
  Data Store Read1/1 -> Logical Operator2/1
  Data Store Read2/1 -> Logical Operator2/2
  Data Store Read3/1 -> Unit Delay2/1
  Data Store Read10/1 -> Unit Delay5/1
  Data Store Read11/1 -> Logical Operator14/1
  Logical Operator8/1 -> Logical Operator10/2
  Data Store Read4/1 -> Logical Operator8/1
  Data Store Read5/1 -> Logical Operator8/2
  Data Store Read14/1 -> Logical Operator14/2
  Logical Operator14/1 -> Logical Operator11/2
  Data Store Read15/1 -> Unit Delay17/1
  Logical Operator16/1 -> Logical Operator15/2
  Data Store Read26/1 -> Unit Delay8/1
  Data Store Read27/1 -> Logical Operator17/2
  Logical Operator3/1 -> Logical Operator18/1
  Logical Operator17/1 -> Logical Operator18/2
  Logical Operator18/1 -> Data Type Conversion2/1
  KL15/1 -> Terminator/1
  Add/1 -> Ecu_St/1
  Data Store Read20/1 -> Unit Delay6/1
  Data Store Read21/1 -> Logical Operator1/2
  Logical Operator19/1 -> Data Type Conversion3/1
  Gain1/1 -> Add/1
  Gain5/1 -> Add/2
  Gain3/1 -> Add/3

== system TM_DynamicModel_Library/DM_Ecu_StBusReq/DM_Ign_Mode ==
  EIS_IgnSwState : Inport
  Constant : Constant  Value=3
  Relational Operator : RelationalOperator  OutDataTypeStr=boolean
  Ign_Mode : Outport
  wires:
  Constant/1 -> Relational Operator/2
  EIS_IgnSwState/1 -> Relational Operator/1
  Relational Operator/1 -> Ign_Mode/1

== system TM_DynamicModel_Library/DM_Eng_Cyc_Time/Counter_RE ==
  Enable : Inport
  Reset : Inport  Port=2
  InitVal : Inport  Port=3
  Add1 : Sum
  Constant1 : Constant
  Switch2 : Switch  Threshold=1
  Switch3 : Switch  Threshold=1
  Unit Delay3 : UnitDelay  SampleTime=-1
  y : Outport  InitialOutput=0
  wires:
  Switch3/1 -> y/1, Unit Delay3/1  "c_k"
  Unit Delay3/1 -> Switch2/3, Add1/1  "c_km1"
  Constant1/1 -> Add1/2
  Add1/1 -> Switch2/1
  Enable/1 -> Switch2/2
  InitVal/1 -> Switch3/1
  Switch2/1 -> Switch3/3
  Reset/1 -> Switch3/2

== system TM_DynamicModel_Library/DM_Eng_Cyc_Time/DM_IgnSwRun_Mode ==
  EIS_IgnSwState : Inport
  Constant : Constant  Value=4
  Relational Operator : RelationalOperator  Operator===  OutDataTypeStr=boolean
  IgnSwRun_Mode : Outport
  wires:
  Constant/1 -> Relational Operator/2
  EIS_IgnSwState/1 -> Relational Operator/1
  Relational Operator/1 -> IgnSwRun_Mode/1  "IgnSwRun_Mode"

== system TM_DynamicModel_Library/DM_Eng_Cyc_Time/EdgeBi ==
  u : Inport
  R : Inport  Port=2
  IV : Inport  Port=3
  Relational Operator : RelationalOperator  Operator=~=  OutDataTypeStr=boolean
  Switch2 : Switch  Threshold=1
  Unit Delay3 : UnitDelay  SampleTime=-1
  y : Outport  InitialOutput=0
  wires:
  Switch2/1 -> Relational Operator/2
  Relational Operator/1 -> y/1  "y_k"
  u/1 -> Unit Delay3/1, Relational Operator/1
  R/1 -> Switch2/2
  Unit Delay3/1 -> Switch2/3  "u_km1"
  IV/1 -> Switch2/1

== system TM_DynamicModel_Library/DM_Eng_Ign_Time/Counter_RE ==
  Enable : Inport
  Reset : Inport  Port=2
  InitVal : Inport  Port=3
  Add1 : Sum
  Constant1 : Constant
  Switch2 : Switch  Threshold=1
  Switch3 : Switch  Threshold=1
  Unit Delay3 : UnitDelay  SampleTime=-1
  y : Outport  InitialOutput=0
  wires:
  Switch3/1 -> y/1, Unit Delay3/1  "c_k"
  Unit Delay3/1 -> Switch2/3, Add1/1  "c_km1"
  Constant1/1 -> Add1/2
  Add1/1 -> Switch2/1
  Enable/1 -> Switch2/2
  InitVal/1 -> Switch3/1
  Switch2/1 -> Switch3/3
  Reset/1 -> Switch3/2

== system TM_DynamicModel_Library/DM_Eng_Ign_Time/DM_Ign_Mode ==
  EIS_IgnSwState : Inport
  Constant : Constant  Value=3
  Relational Operator : RelationalOperator  OutDataTypeStr=boolean
  Ign_Mode : Outport
  wires:
  Constant/1 -> Relational Operator/2
  EIS_IgnSwState/1 -> Relational Operator/1
  Relational Operator/1 -> Ign_Mode/1

== system TM_DynamicModel_Library/DM_Eng_Ign_Time/EdgeBi ==
  u : Inport
  R : Inport  Port=2
  IV : Inport  Port=3
  Relational Operator : RelationalOperator  Operator=~=  OutDataTypeStr=boolean
  Switch2 : Switch  Threshold=1
  Unit Delay3 : UnitDelay  SampleTime=-1
  y : Outport  InitialOutput=0
  wires:
  Switch2/1 -> Relational Operator/2
  Relational Operator/1 -> y/1  "y_k"
  u/1 -> Unit Delay3/1, Relational Operator/1
  R/1 -> Switch2/2
  Unit Delay3/1 -> Switch2/3  "u_km1"
  IV/1 -> Switch2/1

== system TM_DynamicModel_Library/DM_Eng_Run2_Mode/My_SRFF ==
  S : Inport
  R : Inport  Port=2
  Constant : Constant
  Constant1 : Constant  Value=0
  Logical Operator : Logic  Operator=NOT  AllPortsSameDT=off  OutDataTypeStr=boolean
  Switch : Switch  Threshold=1
  Switch1 : Switch  Threshold=1
  Unit Delay : UnitDelay  SampleTime=-1
  Q : Outport
  Not_Q : Outport  Port=2
  wires:
  Unit Delay/1 -> Switch1/3  "q_km1"
  Switch1/1 -> Switch/3
  Constant/1 -> Switch1/1
  Switch/1 -> Logical Operator/1, Q/1, Unit Delay/1  "q_k"
  Constant1/1 -> Switch/1
  R/1 -> Switch/2
  S/1 -> Switch1/2
  Logical Operator/1 -> Not_Q/1

== system TM_DynamicModel_Library/DM_Eng_Run_Time/Counter_RE ==
  Enable : Inport
  Reset : Inport  Port=2
  InitVal : Inport  Port=3
  Add1 : Sum
  Constant1 : Constant
  Switch2 : Switch  Threshold=1
  Switch3 : Switch  Threshold=1
  Unit Delay3 : UnitDelay  SampleTime=-1
  y : Outport  InitialOutput=0
  wires:
  Switch3/1 -> y/1, Unit Delay3/1  "c_k"
  Unit Delay3/1 -> Switch2/3, Add1/1  "c_km1"
  Constant1/1 -> Add1/2
  Add1/1 -> Switch2/1
  Enable/1 -> Switch2/2
  InitVal/1 -> Switch3/1
  Switch2/1 -> Switch3/3
  Reset/1 -> Switch3/2

== system TM_DynamicModel_Library/DM_Eng_Run_Time/Eng_Run2_Mode_Sys ==
  Eng_Spd : Inport
  Compare To Constant : simulink/Logic and Bit Operations/Compare To Constant  relop=>  const=300  OutDataTypeStr=uint8
  Compare To Constant1 : simulink/Logic and Bit Operations/Compare To Constant  relop=<  const=100  OutDataTypeStr=uint8
  My_SRFF : Subsystem
  Terminator : Terminator
  Eng_Run2_Mode : Outport
  wires:
  My_SRFF/1(Q) -> Eng_Run2_Mode/1
  Compare To Constant/1 -> My_SRFF/1(R)
  Compare To Constant1/1 -> My_SRFF/2(S)
  Eng_Spd/1 -> Compare To Constant1/1, Compare To Constant/1
  My_SRFF/2(Not_Q) -> Terminator/1

== system TM_DynamicModel_Library/DM_Eng_Run_Time_ul/Counter_RE ==
  Enable : Inport
  Reset : Inport  Port=2
  InitVal : Inport  Port=3
  Add1 : Sum
  Constant1 : Constant
  Switch2 : Switch  Threshold=1
  Switch3 : Switch  Threshold=1
  Unit Delay3 : UnitDelay  SampleTime=-1
  y : Outport  InitialOutput=0
  wires:
  Reset/1 -> Switch3/2
  Switch2/1 -> Switch3/3
  InitVal/1 -> Switch3/1
  Enable/1 -> Switch2/2
  Add1/1 -> Switch2/1
  Constant1/1 -> Add1/2
  Unit Delay3/1 -> Add1/1, Switch2/3  "c_km1"
  Switch3/1 -> Unit Delay3/1, y/1  "c_k"

== system TM_DynamicModel_Library/DM_HDC_PTReady_Mode/DM_Ign_Mode ==
  EIS_IgnSwState : Inport
  Constant : Constant  Value=3
  Relational Operator : RelationalOperator  OutDataTypeStr=boolean
  Ign_Mode : Outport
  wires:
  Constant/1 -> Relational Operator/2
  EIS_IgnSwState/1 -> Relational Operator/1
  Relational Operator/1 -> Ign_Mode/1

== system TM_DynamicModel_Library/DM_Idle_Mode_Req/DM_APP_Char_out_ub ==
  APP : Inport
  Characterisation : Lookup  InputValues=[0,10,20,30,40,50,60,70,80,90,100]  Table=[0,8,17,26,35,44,59,70,82,91,100]
  APP_Char_out_ub : Outport
  wires:
  APP/1 -> Characterisation/1
  Characterisation/1 -> APP_Char_out_ub/1

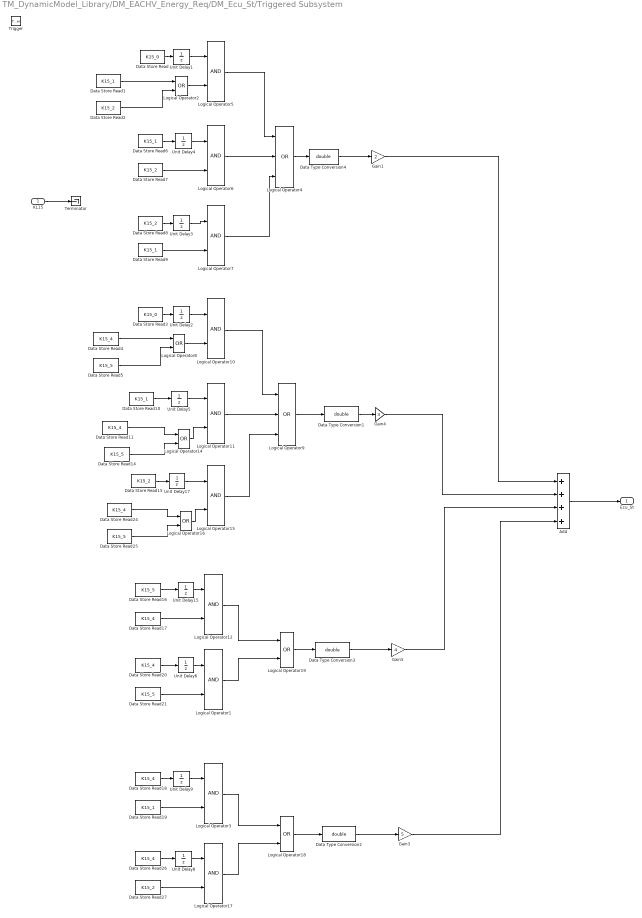
== system TM_DynamicModel_Library/DM_EACHV_Energy_Req/DM_Ecu_St/Triggered Subsystem ==
  KL15 : Inport
  Trigger : TriggerPort  TriggerType=either
  Add : Sum  Inputs=++++
  Data Store Read : DataStoreRead  DataStoreName=K15_0
  Data Store Read{1,6,9..10,19} (5 alike) : DataStoreRead  DataStoreName=K15_1
  Data Store Read{4,11,17..18,20,24,26} (7 alike) : DataStoreRead  DataStoreName=K15_4
  Data Store Read{5,14,16,21,25} (5 alike) : DataStoreRead  DataStoreName=K15_5
  Data Store Read{2,7..8,15,27} (5 alike) : DataStoreRead  DataStoreName=K15_2
  Data Store Read3 : DataStoreRead  DataStoreName=K15_0
  Data Type Conversion{1..4} (4 alike) : DataTypeConversion  OutDataTypeStr=double
  Gain1 : Gain  Gain=2
  Gain3 : Gain  Gain=5
  Gain4 : Gain  Gain=3
  Gain5 : Gain  Gain=4
  Logical Operator{1,3,5..7,10..12,15,17} (10 alike) : Logic  AllPortsSameDT=off  OutDataTypeStr=boolean
  Logical Operator{2,8,14,16,18..19} (6 alike) : Logic  Operator=OR  AllPortsSameDT=off  OutDataTypeStr=boolean
  Logical Operator4 : Logic  Operator=OR  Inputs=3  AllPortsSameDT=off  OutDataTypeStr=boolean
  Logical Operator9 : Logic  Operator=OR  Inputs=3  AllPortsSameDT=off  OutDataTypeStr=boolean
  Terminator : Terminator
  Unit Delay{1..6,8..9,15,17} (10 alike) : UnitDelay  SampleTime=-1
  Ecu_St : Outport
  wires:
  Gain3/1 -> Add/4
  Gain5/1 -> Add/3
  Gain4/1 -> Add/2
  Gain1/1 -> Add/1
  Logical Operator19/1 -> Data Type Conversion3/1
  Logical Operator1/1 -> Logical Operator19/2
  Logical Operator12/1 -> Logical Operator19/1
  Unit Delay6/1 -> Logical Operator1/1
  Data Store Read21/1 -> Logical Operator1/2
  Data Store Read20/1 -> Unit Delay6/1
  Add/1 -> Ecu_St/1
  Unit Delay5/1 -> Logical Operator11/1
  Unit Delay2/1 -> Logical Operator10/1
  Unit Delay3/1 -> Logical Operator7/1
  Unit Delay4/1 -> Logical Operator6/1
  Unit Delay1/1 -> Logical Operator5/1
  KL15/1 -> Terminator/1
  Logical Operator18/1 -> Data Type Conversion2/1
  Logical Operator17/1 -> Logical Operator18/2
  Logical Operator3/1 -> Logical Operator18/1
  Unit Delay8/1 -> Logical Operator17/1
  Unit Delay9/1 -> Logical Operator3/1
  Data Store Read27/1 -> Logical Operator17/2
  Data Store Read26/1 -> Unit Delay8/1
  Unit Delay15/1 -> Logical Operator12/1
  Unit Delay17/1 -> Logical Operator15/1
  Logical Operator15/1 -> Logical Operator9/3
  Logical Operator16/1 -> Logical Operator15/2
  Data Store Read25/1 -> Logical Operator16/2
  Data Store Read24/1 -> Logical Operator16/1
  Data Store Read15/1 -> Unit Delay17/1
  Logical Operator14/1 -> Logical Operator11/2
  Data Store Read14/1 -> Logical Operator14/2
  Data Store Read5/1 -> Logical Operator8/2
  Data Store Read4/1 -> Logical Operator8/1
  Logical Operator8/1 -> Logical Operator10/2
  Data Store Read11/1 -> Logical Operator14/1
  Logical Operator11/1 -> Logical Operator9/2
  Logical Operator10/1 -> Logical Operator9/1
  Data Store Read10/1 -> Unit Delay5/1
  Data Store Read3/1 -> Unit Delay2/1
  Data Store Read2/1 -> Logical Operator2/2
  Data Store Read1/1 -> Logical Operator2/1
  Logical Operator2/1 -> Logical Operator5/2
  Data Store Read7/1 -> Logical Operator6/2
  Data Type Conversion4/1 -> Gain1/1
  Data Type Conversion1/1 -> Gain4/1
  Data Type Conversion3/1 -> Gain5/1
  Data Store Read17/1 -> Logical Operator12/2
  Data Store Read16/1 -> Unit Delay15/1
  Logical Operator9/1 -> Data Type Conversion1/1
  Logical Operator4/1 -> Data Type Conversion4/1
  Logical Operator7/1 -> Logical Operator4/3
  Logical Operator6/1 -> Logical Operator4/2
  Logical Operator5/1 -> Logical Operator4/1
  Data Store Read9/1 -> Logical Operator7/2
  Data Store Read8/1 -> Unit Delay3/1
  Data Store Read6/1 -> Unit Delay4/1
  Data Store Read/1 -> Unit Delay1/1
  Data Type Conversion2/1 -> Gain3/1
  Data Store Read19/1 -> Logical Operator3/2
  Data Store Read18/1 -> Unit Delay9/1

== system TM_DynamicModel_Library/DM_Eng_Run_Time/Eng_Run2_Mode_Sys/My_SRFF ==
  R : Inport
  S : Inport  Port=2
  Constant : Constant
  Constant1 : Constant  Value=0
  Logical Operator : Logic  Operator=NOT  AllPortsSameDT=off  OutDataTypeStr=boolean
  Switch : Switch  Threshold=1
  Switch1 : Switch  Threshold=1
  Unit Delay : UnitDelay  SampleTime=-1
  Q : Outport
  Not_Q : Outport  Port=2
  wires:
  Logical Operator/1 -> Not_Q/1
  S/1 -> Switch1/2
  R/1 -> Switch/2
  Constant1/1 -> Switch/1
  Switch/1 -> Unit Delay/1, Q/1, Logical Operator/1  "q_k"
  Constant/1 -> Switch1/1
  Switch1/1 -> Switch/3
  Unit Delay/1 -> Switch1/3  "q_km1"
